simulink library "relay_PQSPF_lib"  (Simulink 8.1)
settings: Solver=ode45  StartTime=0.0  StopTime=10.0  RelTol=1e-3
libraries: simulink x7
settings Model: Creator=RE25624  LastModifiedBy=ed12083

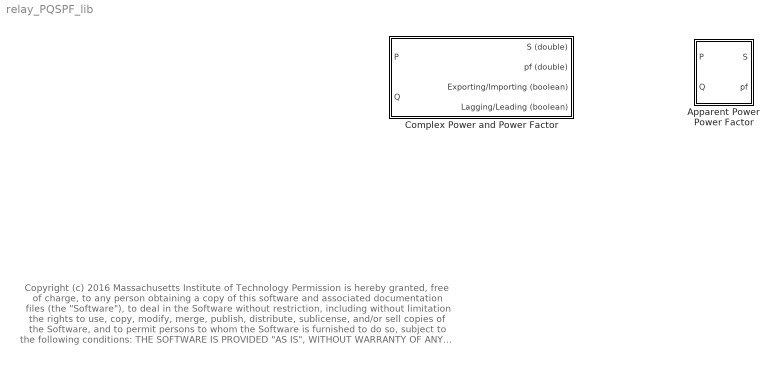
== system relay_PQSPF_lib ==
  note: Copyright (c) 2016 Massachusetts Institute of Technology
      | Permission is hereby granted, free of charge, to any person obtaining a copy of this software and associated documentation files (the "Software"), to deal
      | in the Software without restriction, including without limitation the rights to use, copy, modify, merge, publish, distribute, sublicense, and/or sell copies of the
      | Software, and to permit persons to whom the Software is furnished to do so, subject to the following conditions:
      |
      | THE SOFTWARE IS PROVIDED "AS IS", WITHOUT WARRANTY OF ANY KIND, EXPRESS OR IMPLIED, INCLUDING BUT NOT LIMITED TO THE
      | WARRANTIES OF MERCHANTABILITY, FITNESS FOR A PARTICULAR PURPOSE AND NONINFRINGEMENT. IN NO EVENT SHALL THE AUTHORS
      | OR COPYRIGHT HOLDERS BE LIABLE FOR ANY CLAIM, DAMAGES OR OTHER LIABILITY, WHETHER IN AN ACTION OF CONTRACT, TORT OR
      | OTHERWISE, ARISING FROM, OUT OF OR IN CONNECTION WITH THE SOFTWARE OR THE USE OR OTHER DEALINGS IN THE SOFTWARE.
  Apparent Power Power Factor : Subsystem
  Complex Power and Power Factor : Subsystem

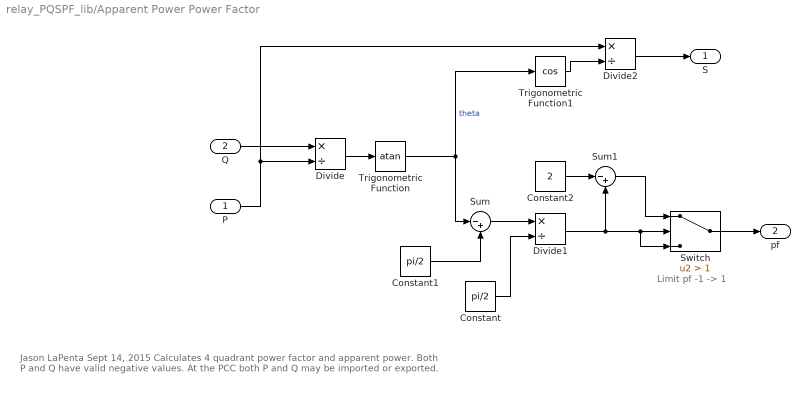
== system relay_PQSPF_lib/Apparent Power Power Factor ==
  note: Jason LaPenta
      | Sept 14, 2015
      |
      | Calculates 4 quadrant power factor and apparent power.
      | Both P and Q have valid negative values. At the PCC
      | both P and Q may be imported or exported.
  note: Limit pf -1 -> 1
  P : Inport
  Q : Inport  Port=2
  Constant : Constant  Value=pi/2
  Constant1 : Constant  Value=pi/2
  Constant2 : Constant  Value=2
  Divide : Product  Inputs=*/
  Divide1 : Product  Inputs=*/
  Divide2 : Product  Inputs=*/
  Sum : Sum  Inputs=|-+
  Sum1 : Sum  Inputs=|-+
  Switch : Switch  Criteria=u2 > Threshold  Threshold=1
  Trigonometric Function : Trigonometry  Operator=atan
  Trigonometric Function1 : Trigonometry  Operator=cos
  S : Outport
  pf : Outport  Port=2
  wires:
  Q/1 -> Divide/1
  P/1 -> Divide/2, Divide2/1
  Divide/1 -> Trigonometric Function/1
  Trigonometric Function/1 -> Trigonometric Function1/1, Sum/1  "theta"
  Constant/1 -> Divide1/2
  Trigonometric Function1/1 -> Divide2/2
  Divide2/1 -> S/1
  Constant1/1 -> Sum/2
  Sum/1 -> Divide1/1
  Divide1/1 -> Sum1/2, Switch/2, Switch/3
  Sum1/1 -> Switch/1
  Constant2/1 -> Sum1/1
  Switch/1 -> pf/1

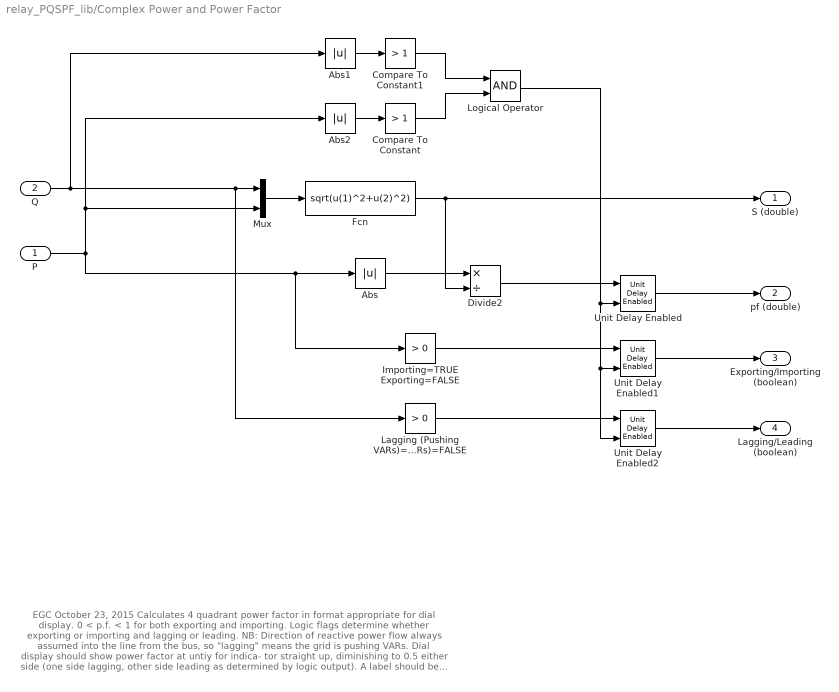
== system relay_PQSPF_lib/Complex Power and Power Factor ==
  note: EGC
      | October 23, 2015
      |
      | Calculates 4 quadrant power factor in format appropriate
      | for dial display.  0 < p.f. < 1 for both exporting and
      | importing.  Logic flags determine whether exporting or
      | importing and lagging or leading.  NB:  Direction of
      | reactive power flow always assumed into the line from the
      | bus, so "lagging" means the grid is pushing VARs.
      |
      | Dial display should show power factor at untiy for indica-
      | tor straight up, diminishing to 0.5 either side (one side
      | lagging, other side leading as determined by logic output).
      | A label should be used to display EXPORTING or IMPORTING
      | based on logic output.
  P : Inport
  Q : Inport  Port=2
  Abs : Abs
  Abs1 : Abs
  Abs2 : Abs
  Compare To Constant : simulink/Logic and Bit Operations/Compare To Constant  relop=>  const=1  OutDataTypeStr=uint8
  Compare To Constant1 : simulink/Logic and Bit Operations/Compare To Constant  relop=>  const=1  OutDataTypeStr=uint8
  Divide2 : Product  Inputs=*/
  Fcn : Fcn  Expr=sqrt(u(1)^2+u(2)^2)
  Importing=TRUE Exporting=FALSE : simulink/Logic and Bit Operations/Compare To Constant  relop=>  const=0  OutDataTypeStr=boolean
  Lagging (Pushing VARs)=TRUE Leading (Pulling VARs)=FALSE : simulink/Logic and Bit Operations/Compare To Constant  relop=>  const=0  OutDataTypeStr=boolean
  Logical Operator : Logic  AllPortsSameDT=off  OutDataTypeStr=boolean
  Mux : Mux  Inputs=2
  Unit Delay Enabled : simulink/Additional Math & Discrete/Additional Discrete/Unit Delay Enabled  vinit=1  tsamp=-1
  Unit Delay Enabled1 : simulink/Additional Math & Discrete/Additional Discrete/Unit Delay Enabled  vinit=1  tsamp=-1
  Unit Delay Enabled2 : simulink/Additional Math & Discrete/Additional Discrete/Unit Delay Enabled  vinit=1  tsamp=-1
  S (double) : Outport
  pf (double) : Outport  Port=2
  Exporting/Importing (boolean) : Outport  Port=3
  Lagging/Leading (boolean) : Outport  Port=4
  wires:
  Logical Operator/1 -> Unit Delay Enabled2/2, Unit Delay Enabled1/2, Unit Delay Enabled/2
  Compare To Constant/1 -> Logical Operator/2
  Compare To Constant1/1 -> Logical Operator/1
  Abs1/1 -> Compare To Constant1/1
  Abs2/1 -> Compare To Constant/1
  Unit Delay Enabled2/1 -> Lagging/Leading (boolean)/1
  Lagging (Pushing VARs)=TRUE Leading (Pulling VARs)=FALSE/1 -> Unit Delay Enabled2/1
  Unit Delay Enabled1/1 -> Exporting/Importing (boolean)/1
  Importing=TRUE Exporting=FALSE/1 -> Unit Delay Enabled1/1
  Unit Delay Enabled/1 -> pf (double)/1
  Divide2/1 -> Unit Delay Enabled/1
  Abs/1 -> Divide2/1
  Mux/1 -> Fcn/1
  Q/1 -> Abs1/1, Lagging (Pushing VARs)=TRUE Leading (Pulling VARs)=FALSE/1, Mux/1
  P/1 -> Abs2/1, Mux/2, Importing=TRUE Exporting=FALSE/1, Abs/1
  Fcn/1 -> S (double)/1, Divide2/2
